simulink model "ControlSystemPID"  (R2020b)
settings: Solver=ode23s  StartTime=0.0  StopTime=3.5  MaxStep=0.06  RelTol=1e-3
model workspace: external: MATLAB File C:\Users\User\Aalborg Universitet\ROB 3 - General\P3\Solidworks_files\SimScapeV4\TotalAssemblyV4_DataFile.m (data not in the file)
values from neighbouring files (symbols this model uses):
  Ki = 10    [Data.m]
  Kp = 200    [Data.m]
  Kv = 127    [Data.m]
undefined symbols (not defined in the file or in its folder): smiData, X, Y, Z
libraries: sm_lib x112, nesl_utility x16, simulink_extras x9, pid_lib x1
(part 3 of 3)

== system ControlSystemPID/Body3_3_RIGID/Finger_2_RIGID ==
  ReferenceFrame : sm_lib/Frames and Transforms/Reference Frame
  Solid : sm_lib/Body Elements/File Solid  ExtGeomFileName=Finger_Default_sldprt.STEP  UnitType=FromFile  ExtGeomFileUnits=m  StepReaderType=HEX  ExportConvexHullGeometry=off  InertiaType=Custom  Mass=smiData.Solid(16).mass  MassUnits=kg  CenterOfMass=smiData.Solid(16).CoM  CenterOfMassUnits=mm  MomentsOfInertia=smiData.Solid(16).MoI  MomentsOfInertiaUnits=kg*mm^2  ProductsOfInertia=smiData.Solid(16).PoI  ProductsOfInertiaUnits=kg*mm^2  BasedOnType=DensityFromFile  Density=1000  DensityUnits=kg/m^3  DoExposeReferenceFrame=on  SerializedFrames=<Frames/>  GraphicType=FromGeometry  MarkerShape=Sphere  MarkerSize=10  GraphicVisPropType=SimpleVisualProperties  GraphicDiffuseColor=smiData.Solid(16).color  GraphicSpecularColor=[0.5 0.5 0.5 1.0]  GraphicAmbientColor=[0.15 0.15 0.15 1.0]  GraphicEmissiveColor=[0.0 0.0 0.0 1.0]  GraphicShininess=75  GraphicOpacity=smiData.Solid(16).opacity
  F : PMIOPort  Side=Left
  connections:
  Solid/RConn1 -- ReferenceFrame/RConn1 -- F/RConn1

== system ControlSystemPID/Body3_3_RIGID/Link_2_1_RIGID ==
  ReferenceFrame : sm_lib/Frames and Transforms/Reference Frame
  Solid : sm_lib/Body Elements/File Solid  ExtGeomFileName=Link-2_Default_sldprt.STEP  UnitType=FromFile  ExtGeomFileUnits=m  StepReaderType=HEX  ExportConvexHullGeometry=off  InertiaType=Custom  Mass=smiData.Solid(11).mass  MassUnits=kg  CenterOfMass=smiData.Solid(11).CoM  CenterOfMassUnits=mm  MomentsOfInertia=smiData.Solid(11).MoI  MomentsOfInertiaUnits=kg*mm^2  ProductsOfInertia=smiData.Solid(11).PoI  ProductsOfInertiaUnits=kg*mm^2  BasedOnType=DensityFromFile  Density=1000  DensityUnits=kg/m^3  DoExposeReferenceFrame=on  SerializedFrames=<Frames/>  GraphicType=FromGeometry  MarkerShape=Sphere  MarkerSize=10  GraphicVisPropType=SimpleVisualProperties  GraphicDiffuseColor=smiData.Solid(11).color  GraphicSpecularColor=[0.5 0.5 0.5 1.0]  GraphicAmbientColor=[0.15 0.15 0.15 1.0]  GraphicEmissiveColor=[0.0 0.0 0.0 1.0]  GraphicShininess=75  GraphicOpacity=smiData.Solid(11).opacity
  F : PMIOPort  Side=Left
  connections:
  Solid/RConn1 -- ReferenceFrame/RConn1 -- F/RConn1

== system ControlSystemPID/Body3_3_RIGID/Link_plate_1_RIGID ==
  ReferenceFrame : sm_lib/Frames and Transforms/Reference Frame
  Solid : sm_lib/Body Elements/File Solid  ExtGeomFileName=Link-plate_Default_sldprt.STEP  UnitType=FromFile  ExtGeomFileUnits=m  StepReaderType=HEX  ExportConvexHullGeometry=off  InertiaType=Custom  Mass=smiData.Solid(3).mass  MassUnits=kg  CenterOfMass=smiData.Solid(3).CoM  CenterOfMassUnits=mm  MomentsOfInertia=smiData.Solid(3).MoI  MomentsOfInertiaUnits=kg*mm^2  ProductsOfInertia=smiData.Solid(3).PoI  ProductsOfInertiaUnits=kg*mm^2  BasedOnType=DensityFromFile  Density=1000  DensityUnits=kg/m^3  DoExposeReferenceFrame=on  SerializedFrames=<Frames/>  GraphicType=FromGeometry  MarkerShape=Sphere  MarkerSize=10  GraphicVisPropType=SimpleVisualProperties  GraphicDiffuseColor=smiData.Solid(3).color  GraphicSpecularColor=[0.5 0.5 0.5 1.0]  GraphicAmbientColor=[0.15 0.15 0.15 1.0]  GraphicEmissiveColor=[0.0 0.0 0.0 1.0]  GraphicShininess=75  GraphicOpacity=smiData.Solid(3).opacity
  F : PMIOPort  Side=Left
  connections:
  Solid/RConn1 -- ReferenceFrame/RConn1 -- F/RConn1

== system ControlSystemPID/Body3_3_RIGID/MX_28T_1_RIGID ==
  ReferenceFrame : sm_lib/Frames and Transforms/Reference Frame
  Solid : sm_lib/Body Elements/File Solid  ExtGeomFileName=MX-28T_Default_sldprt.STEP  UnitType=FromFile  ExtGeomFileUnits=m  StepReaderType=HEX  ExportConvexHullGeometry=off  InertiaType=Custom  Mass=smiData.Solid(13).mass  MassUnits=kg  CenterOfMass=smiData.Solid(13).CoM  CenterOfMassUnits=mm  MomentsOfInertia=smiData.Solid(13).MoI  MomentsOfInertiaUnits=kg*mm^2  ProductsOfInertia=smiData.Solid(13).PoI  ProductsOfInertiaUnits=kg*mm^2  BasedOnType=DensityFromFile  Density=1000  DensityUnits=kg/m^3  DoExposeReferenceFrame=on  SerializedFrames=<Frames/>  GraphicType=FromGeometry  MarkerShape=Sphere  MarkerSize=10  GraphicVisPropType=SimpleVisualProperties  GraphicDiffuseColor=smiData.Solid(13).color  GraphicSpecularColor=[0.5 0.5 0.5 1.0]  GraphicAmbientColor=[0.15 0.15 0.15 1.0]  GraphicEmissiveColor=[0.0 0.0 0.0 1.0]  GraphicShininess=75  GraphicOpacity=smiData.Solid(13).opacity
  F : PMIOPort  Side=Left
  connections:
  Solid/RConn1 -- ReferenceFrame/RConn1 -- F/RConn1

== system ControlSystemPID/Body3_3_RIGID/MX_28T_2_RIGID ==
  ReferenceFrame : sm_lib/Frames and Transforms/Reference Frame
  Solid : sm_lib/Body Elements/File Solid  ExtGeomFileName=MX-28T_Default_sldprt.STEP  UnitType=FromFile  ExtGeomFileUnits=m  StepReaderType=HEX  ExportConvexHullGeometry=off  InertiaType=Custom  Mass=smiData.Solid(13).mass  MassUnits=kg  CenterOfMass=smiData.Solid(13).CoM  CenterOfMassUnits=mm  MomentsOfInertia=smiData.Solid(13).MoI  MomentsOfInertiaUnits=kg*mm^2  ProductsOfInertia=smiData.Solid(13).PoI  ProductsOfInertiaUnits=kg*mm^2  BasedOnType=DensityFromFile  Density=1000  DensityUnits=kg/m^3  DoExposeReferenceFrame=on  SerializedFrames=<Frames/>  GraphicType=FromGeometry  MarkerShape=Sphere  MarkerSize=10  GraphicVisPropType=SimpleVisualProperties  GraphicDiffuseColor=smiData.Solid(13).color  GraphicSpecularColor=[0.5 0.5 0.5 1.0]  GraphicAmbientColor=[0.15 0.15 0.15 1.0]  GraphicEmissiveColor=[0.0 0.0 0.0 1.0]  GraphicShininess=75  GraphicOpacity=smiData.Solid(13).opacity
  F : PMIOPort  Side=Left
  connections:
  Solid/RConn1 -- ReferenceFrame/RConn1 -- F/RConn1

== system ControlSystemPID/Body3_3_RIGID/MX_28T_Link_1_RIGID ==
  ReferenceFrame : sm_lib/Frames and Transforms/Reference Frame
  Solid : sm_lib/Body Elements/File Solid  ExtGeomFileName=MX-28T-Link_Default_sldprt.STEP  UnitType=FromFile  ExtGeomFileUnits=m  StepReaderType=HEX  ExportConvexHullGeometry=off  InertiaType=Custom  Mass=smiData.Solid(17).mass  MassUnits=kg  CenterOfMass=smiData.Solid(17).CoM  CenterOfMassUnits=mm  MomentsOfInertia=smiData.Solid(17).MoI  MomentsOfInertiaUnits=kg*mm^2  ProductsOfInertia=smiData.Solid(17).PoI  ProductsOfInertiaUnits=kg*mm^2  BasedOnType=DensityFromFile  Density=1000  DensityUnits=kg/m^3  DoExposeReferenceFrame=on  SerializedFrames=<Frames/>  GraphicType=FromGeometry  MarkerShape=Sphere  MarkerSize=10  GraphicVisPropType=SimpleVisualProperties  GraphicDiffuseColor=smiData.Solid(17).color  GraphicSpecularColor=[0.5 0.5 0.5 1.0]  GraphicAmbientColor=[0.15 0.15 0.15 1.0]  GraphicEmissiveColor=[0.0 0.0 0.0 1.0]  GraphicShininess=75  GraphicOpacity=smiData.Solid(17).opacity
  F : PMIOPort  Side=Left
  connections:
  Solid/RConn1 -- ReferenceFrame/RConn1 -- F/RConn1

== system ControlSystemPID/Body3_3_RIGID/MX_28T_Link_2_RIGID ==
  ReferenceFrame : sm_lib/Frames and Transforms/Reference Frame
  Solid : sm_lib/Body Elements/File Solid  ExtGeomFileName=MX-28T-Link_Default_sldprt.STEP  UnitType=FromFile  ExtGeomFileUnits=m  StepReaderType=HEX  ExportConvexHullGeometry=off  InertiaType=Custom  Mass=smiData.Solid(17).mass  MassUnits=kg  CenterOfMass=smiData.Solid(17).CoM  CenterOfMassUnits=mm  MomentsOfInertia=smiData.Solid(17).MoI  MomentsOfInertiaUnits=kg*mm^2  ProductsOfInertia=smiData.Solid(17).PoI  ProductsOfInertiaUnits=kg*mm^2  BasedOnType=DensityFromFile  Density=1000  DensityUnits=kg/m^3  DoExposeReferenceFrame=on  SerializedFrames=<Frames/>  GraphicType=FromGeometry  MarkerShape=Sphere  MarkerSize=10  GraphicVisPropType=SimpleVisualProperties  GraphicDiffuseColor=smiData.Solid(17).color  GraphicSpecularColor=[0.5 0.5 0.5 1.0]  GraphicAmbientColor=[0.15 0.15 0.15 1.0]  GraphicEmissiveColor=[0.0 0.0 0.0 1.0]  GraphicShininess=75  GraphicOpacity=smiData.Solid(17).opacity
  F : PMIOPort  Side=Left
  connections:
  Solid/RConn1 -- ReferenceFrame/RConn1 -- F/RConn1

== system ControlSystemPID/Body3_3_RIGID/Servo_Disc_1_RIGID ==
  ReferenceFrame : sm_lib/Frames and Transforms/Reference Frame
  Solid : sm_lib/Body Elements/File Solid  ExtGeomFileName=Servo-Disc_Default_sldprt.STEP  UnitType=FromFile  ExtGeomFileUnits=m  StepReaderType=HEX  ExportConvexHullGeometry=off  InertiaType=Custom  Mass=smiData.Solid(2).mass  MassUnits=kg  CenterOfMass=smiData.Solid(2).CoM  CenterOfMassUnits=mm  MomentsOfInertia=smiData.Solid(2).MoI  MomentsOfInertiaUnits=kg*mm^2  ProductsOfInertia=smiData.Solid(2).PoI  ProductsOfInertiaUnits=kg*mm^2  BasedOnType=DensityFromFile  Density=1000  DensityUnits=kg/m^3  DoExposeReferenceFrame=on  SerializedFrames=<Frames/>  GraphicType=FromGeometry  MarkerShape=Sphere  MarkerSize=10  GraphicVisPropType=SimpleVisualProperties  GraphicDiffuseColor=smiData.Solid(2).color  GraphicSpecularColor=[0.5 0.5 0.5 1.0]  GraphicAmbientColor=[0.15 0.15 0.15 1.0]  GraphicEmissiveColor=[0.0 0.0 0.0 1.0]  GraphicShininess=75  GraphicOpacity=smiData.Solid(2).opacity
  F : PMIOPort  Side=Left
  connections:
  Solid/RConn1 -- ReferenceFrame/RConn1 -- F/RConn1

== system ControlSystemPID/Body3_3_RIGID/Servo_Disc_2_RIGID ==
  ReferenceFrame : sm_lib/Frames and Transforms/Reference Frame
  Solid : sm_lib/Body Elements/File Solid  ExtGeomFileName=Servo-Disc_Default_sldprt.STEP  UnitType=FromFile  ExtGeomFileUnits=m  StepReaderType=HEX  ExportConvexHullGeometry=off  InertiaType=Custom  Mass=smiData.Solid(2).mass  MassUnits=kg  CenterOfMass=smiData.Solid(2).CoM  CenterOfMassUnits=mm  MomentsOfInertia=smiData.Solid(2).MoI  MomentsOfInertiaUnits=kg*mm^2  ProductsOfInertia=smiData.Solid(2).PoI  ProductsOfInertiaUnits=kg*mm^2  BasedOnType=DensityFromFile  Density=1000  DensityUnits=kg/m^3  DoExposeReferenceFrame=on  SerializedFrames=<Frames/>  GraphicType=FromGeometry  MarkerShape=Sphere  MarkerSize=10  GraphicVisPropType=SimpleVisualProperties  GraphicDiffuseColor=smiData.Solid(2).color  GraphicSpecularColor=[0.5 0.5 0.5 1.0]  GraphicAmbientColor=[0.15 0.15 0.15 1.0]  GraphicEmissiveColor=[0.0 0.0 0.0 1.0]  GraphicShininess=75  GraphicOpacity=smiData.Solid(2).opacity
  F : PMIOPort  Side=Left
  connections:
  Solid/RConn1 -- ReferenceFrame/RConn1 -- F/RConn1

== system ControlSystemPID/Body3_3_RIGID/Servo_Disc_3_RIGID ==
  ReferenceFrame : sm_lib/Frames and Transforms/Reference Frame
  Solid : sm_lib/Body Elements/File Solid  ExtGeomFileName=Servo-Disc_Default_sldprt.STEP  UnitType=FromFile  ExtGeomFileUnits=m  StepReaderType=HEX  ExportConvexHullGeometry=off  InertiaType=Custom  Mass=smiData.Solid(2).mass  MassUnits=kg  CenterOfMass=smiData.Solid(2).CoM  CenterOfMassUnits=mm  MomentsOfInertia=smiData.Solid(2).MoI  MomentsOfInertiaUnits=kg*mm^2  ProductsOfInertia=smiData.Solid(2).PoI  ProductsOfInertiaUnits=kg*mm^2  BasedOnType=DensityFromFile  Density=1000  DensityUnits=kg/m^3  DoExposeReferenceFrame=on  SerializedFrames=<Frames/>  GraphicType=FromGeometry  MarkerShape=Sphere  MarkerSize=10  GraphicVisPropType=SimpleVisualProperties  GraphicDiffuseColor=smiData.Solid(2).color  GraphicSpecularColor=[0.5 0.5 0.5 1.0]  GraphicAmbientColor=[0.15 0.15 0.15 1.0]  GraphicEmissiveColor=[0.0 0.0 0.0 1.0]  GraphicShininess=75  GraphicOpacity=smiData.Solid(2).opacity
  F : PMIOPort  Side=Left
  connections:
  Solid/RConn1 -- ReferenceFrame/RConn1 -- F/RConn1

== system ControlSystemPID/Body3_3_RIGID/Servo_Disc_4_RIGID ==
  ReferenceFrame : sm_lib/Frames and Transforms/Reference Frame
  Solid : sm_lib/Body Elements/File Solid  ExtGeomFileName=Servo-Disc_Default_sldprt.STEP  UnitType=FromFile  ExtGeomFileUnits=m  StepReaderType=HEX  ExportConvexHullGeometry=off  InertiaType=Custom  Mass=smiData.Solid(2).mass  MassUnits=kg  CenterOfMass=smiData.Solid(2).CoM  CenterOfMassUnits=mm  MomentsOfInertia=smiData.Solid(2).MoI  MomentsOfInertiaUnits=kg*mm^2  ProductsOfInertia=smiData.Solid(2).PoI  ProductsOfInertiaUnits=kg*mm^2  BasedOnType=DensityFromFile  Density=1000  DensityUnits=kg/m^3  DoExposeReferenceFrame=on  SerializedFrames=<Frames/>  GraphicType=FromGeometry  MarkerShape=Sphere  MarkerSize=10  GraphicVisPropType=SimpleVisualProperties  GraphicDiffuseColor=smiData.Solid(2).color  GraphicSpecularColor=[0.5 0.5 0.5 1.0]  GraphicAmbientColor=[0.15 0.15 0.15 1.0]  GraphicEmissiveColor=[0.0 0.0 0.0 1.0]  GraphicShininess=75  GraphicOpacity=smiData.Solid(2).opacity
  F : PMIOPort  Side=Left
  connections:
  Solid/RConn1 -- ReferenceFrame/RConn1 -- F/RConn1

== system ControlSystemPID/Body3_3_RIGID/Servo_Disc_5_RIGID ==
  ReferenceFrame : sm_lib/Frames and Transforms/Reference Frame
  Solid : sm_lib/Body Elements/File Solid  ExtGeomFileName=Servo-Disc_Default_sldprt.STEP  UnitType=FromFile  ExtGeomFileUnits=m  StepReaderType=HEX  ExportConvexHullGeometry=off  InertiaType=Custom  Mass=smiData.Solid(2).mass  MassUnits=kg  CenterOfMass=smiData.Solid(2).CoM  CenterOfMassUnits=mm  MomentsOfInertia=smiData.Solid(2).MoI  MomentsOfInertiaUnits=kg*mm^2  ProductsOfInertia=smiData.Solid(2).PoI  ProductsOfInertiaUnits=kg*mm^2  BasedOnType=DensityFromFile  Density=1000  DensityUnits=kg/m^3  DoExposeReferenceFrame=on  SerializedFrames=<Frames/>  GraphicType=FromGeometry  MarkerShape=Sphere  MarkerSize=10  GraphicVisPropType=SimpleVisualProperties  GraphicDiffuseColor=smiData.Solid(2).color  GraphicSpecularColor=[0.5 0.5 0.5 1.0]  GraphicAmbientColor=[0.15 0.15 0.15 1.0]  GraphicEmissiveColor=[0.0 0.0 0.0 1.0]  GraphicShininess=75  GraphicOpacity=smiData.Solid(2).opacity
  F : PMIOPort  Side=Left
  connections:
  Solid/RConn1 -- ReferenceFrame/RConn1 -- F/RConn1

== system ControlSystemPID/Body3_3_RIGID/Servo_Disc_6_RIGID ==
  ReferenceFrame : sm_lib/Frames and Transforms/Reference Frame
  Solid : sm_lib/Body Elements/File Solid  ExtGeomFileName=Servo-Disc_Default_sldprt.STEP  UnitType=FromFile  ExtGeomFileUnits=m  StepReaderType=HEX  ExportConvexHullGeometry=off  InertiaType=Custom  Mass=smiData.Solid(2).mass  MassUnits=kg  CenterOfMass=smiData.Solid(2).CoM  CenterOfMassUnits=mm  MomentsOfInertia=smiData.Solid(2).MoI  MomentsOfInertiaUnits=kg*mm^2  ProductsOfInertia=smiData.Solid(2).PoI  ProductsOfInertiaUnits=kg*mm^2  BasedOnType=DensityFromFile  Density=1000  DensityUnits=kg/m^3  DoExposeReferenceFrame=on  SerializedFrames=<Frames/>  GraphicType=FromGeometry  MarkerShape=Sphere  MarkerSize=10  GraphicVisPropType=SimpleVisualProperties  GraphicDiffuseColor=smiData.Solid(2).color  GraphicSpecularColor=[0.5 0.5 0.5 1.0]  GraphicAmbientColor=[0.15 0.15 0.15 1.0]  GraphicEmissiveColor=[0.0 0.0 0.0 1.0]  GraphicShininess=75  GraphicOpacity=smiData.Solid(2).opacity
  F : PMIOPort  Side=Left
  connections:
  Solid/RConn1 -- ReferenceFrame/RConn1 -- F/RConn1

== system ControlSystemPID/Body3_3_RIGID/Servo_disc_link_MX_28T_1_RIGID ==
  ReferenceFrame : sm_lib/Frames and Transforms/Reference Frame
  Solid : sm_lib/Body Elements/File Solid  ExtGeomFileName=Servo-disc-link_MX-28T_Default_sldprt.STEP  UnitType=FromFile  ExtGeomFileUnits=m  StepReaderType=HEX  ExportConvexHullGeometry=off  InertiaType=Custom  Mass=smiData.Solid(15).mass  MassUnits=kg  CenterOfMass=smiData.Solid(15).CoM  CenterOfMassUnits=mm  MomentsOfInertia=smiData.Solid(15).MoI  MomentsOfInertiaUnits=kg*mm^2  ProductsOfInertia=smiData.Solid(15).PoI  ProductsOfInertiaUnits=kg*mm^2  BasedOnType=DensityFromFile  Density=1000  DensityUnits=kg/m^3  DoExposeReferenceFrame=on  SerializedFrames=<Frames/>  GraphicType=FromGeometry  MarkerShape=Sphere  MarkerSize=10  GraphicVisPropType=SimpleVisualProperties  GraphicDiffuseColor=smiData.Solid(15).color  GraphicSpecularColor=[0.5 0.5 0.5 1.0]  GraphicAmbientColor=[0.15 0.15 0.15 1.0]  GraphicEmissiveColor=[0.0 0.0 0.0 1.0]  GraphicShininess=75  GraphicOpacity=smiData.Solid(15).opacity
  F : PMIOPort  Side=Left
  connections:
  Solid/RConn1 -- ReferenceFrame/RConn1 -- F/RConn1

== system ControlSystemPID/Body3_3_RIGID/Servo_disc_link_MX_28T_2_RIGID ==
  ReferenceFrame : sm_lib/Frames and Transforms/Reference Frame
  Solid : sm_lib/Body Elements/File Solid  ExtGeomFileName=Servo-disc-link_MX-28T_Default_sldprt.STEP  UnitType=FromFile  ExtGeomFileUnits=m  StepReaderType=HEX  ExportConvexHullGeometry=off  InertiaType=Custom  Mass=smiData.Solid(15).mass  MassUnits=kg  CenterOfMass=smiData.Solid(15).CoM  CenterOfMassUnits=mm  MomentsOfInertia=smiData.Solid(15).MoI  MomentsOfInertiaUnits=kg*mm^2  ProductsOfInertia=smiData.Solid(15).PoI  ProductsOfInertiaUnits=kg*mm^2  BasedOnType=DensityFromFile  Density=1000  DensityUnits=kg/m^3  DoExposeReferenceFrame=on  SerializedFrames=<Frames/>  GraphicType=FromGeometry  MarkerShape=Sphere  MarkerSize=10  GraphicVisPropType=SimpleVisualProperties  GraphicDiffuseColor=smiData.Solid(15).color  GraphicSpecularColor=[0.5 0.5 0.5 1.0]  GraphicAmbientColor=[0.15 0.15 0.15 1.0]  GraphicEmissiveColor=[0.0 0.0 0.0 1.0]  GraphicShininess=75  GraphicOpacity=smiData.Solid(15).opacity
  F : PMIOPort  Side=Left
  connections:
  Solid/RConn1 -- ReferenceFrame/RConn1 -- F/RConn1

== system ControlSystemPID/Body3_3_RIGID/Servo_disc_link_MX_64T_1_RIGID ==
  ReferenceFrame : sm_lib/Frames and Transforms/Reference Frame
  Solid : sm_lib/Body Elements/File Solid  ExtGeomFileName=Servo-disc-link_MX-64T_Default_sldprt.STEP  UnitType=FromFile  ExtGeomFileUnits=m  StepReaderType=HEX  ExportConvexHullGeometry=off  InertiaType=Custom  Mass=smiData.Solid(12).mass  MassUnits=kg  CenterOfMass=smiData.Solid(12).CoM  CenterOfMassUnits=mm  MomentsOfInertia=smiData.Solid(12).MoI  MomentsOfInertiaUnits=kg*mm^2  ProductsOfInertia=smiData.Solid(12).PoI  ProductsOfInertiaUnits=kg*mm^2  BasedOnType=DensityFromFile  Density=1000  DensityUnits=kg/m^3  DoExposeReferenceFrame=on  SerializedFrames=<Frames/>  GraphicType=FromGeometry  MarkerShape=Sphere  MarkerSize=10  GraphicVisPropType=SimpleVisualProperties  GraphicDiffuseColor=smiData.Solid(12).color  GraphicSpecularColor=[0.5 0.5 0.5 1.0]  GraphicAmbientColor=[0.15 0.15 0.15 1.0]  GraphicEmissiveColor=[0.0 0.0 0.0 1.0]  GraphicShininess=75  GraphicOpacity=smiData.Solid(12).opacity
  F : PMIOPort  Side=Left
  connections:
  Solid/RConn1 -- ReferenceFrame/RConn1 -- F/RConn1

== system ControlSystemPID/Body3_3_RIGID/Servo_link_link_MX_28T_4_RIGID ==
  ReferenceFrame : sm_lib/Frames and Transforms/Reference Frame
  Solid : sm_lib/Body Elements/File Solid  ExtGeomFileName=Servo-link-link_MX-28T_Default_sldprt.STEP  UnitType=FromFile  ExtGeomFileUnits=m  StepReaderType=HEX  ExportConvexHullGeometry=off  InertiaType=Custom  Mass=smiData.Solid(14).mass  MassUnits=kg  CenterOfMass=smiData.Solid(14).CoM  CenterOfMassUnits=mm  MomentsOfInertia=smiData.Solid(14).MoI  MomentsOfInertiaUnits=kg*mm^2  ProductsOfInertia=smiData.Solid(14).PoI  ProductsOfInertiaUnits=kg*mm^2  BasedOnType=DensityFromFile  Density=1000  DensityUnits=kg/m^3  DoExposeReferenceFrame=on  SerializedFrames=<Frames/>  GraphicType=FromGeometry  MarkerShape=Sphere  MarkerSize=10  GraphicVisPropType=SimpleVisualProperties  GraphicDiffuseColor=smiData.Solid(14).color  GraphicSpecularColor=[0.5 0.5 0.5 1.0]  GraphicAmbientColor=[0.15 0.15 0.15 1.0]  GraphicEmissiveColor=[0.0 0.0 0.0 1.0]  GraphicShininess=75  GraphicOpacity=smiData.Solid(14).opacity
  F : PMIOPort  Side=Left
  connections:
  Solid/RConn1 -- ReferenceFrame/RConn1 -- F/RConn1

== system ControlSystemPID/TableAssembly_2_RIGID/Base_1_RIGID ==
  ReferenceFrame : sm_lib/Frames and Transforms/Reference Frame
  Solid : sm_lib/Body Elements/File Solid  ExtGeomFileName=Base_Default_sldprt.STEP  UnitType=FromFile  ExtGeomFileUnits=m  StepReaderType=HEX  ExportConvexHullGeometry=off  InertiaType=Custom  Mass=smiData.Solid(7).mass  MassUnits=kg  CenterOfMass=smiData.Solid(7).CoM  CenterOfMassUnits=mm  MomentsOfInertia=smiData.Solid(7).MoI  MomentsOfInertiaUnits=kg*mm^2  ProductsOfInertia=smiData.Solid(7).PoI  ProductsOfInertiaUnits=kg*mm^2  BasedOnType=DensityFromFile  Density=1000  DensityUnits=kg/m^3  DoExposeReferenceFrame=on  SerializedFrames=<Frames/>  GraphicType=FromGeometry  MarkerShape=Sphere  MarkerSize=10  GraphicVisPropType=SimpleVisualProperties  GraphicDiffuseColor=smiData.Solid(7).color  GraphicSpecularColor=[0.5 0.5 0.5 1.0]  GraphicAmbientColor=[0.15 0.15 0.15 1.0]  GraphicEmissiveColor=[0.0 0.0 0.0 1.0]  GraphicShininess=75  GraphicOpacity=smiData.Solid(7).opacity
  F : PMIOPort  Side=Left
  connections:
  Solid/RConn1 -- ReferenceFrame/RConn1 -- F/RConn1

== system ControlSystemPID/TableAssembly_2_RIGID/MX_64T_1_RIGID ==
  ReferenceFrame : sm_lib/Frames and Transforms/Reference Frame
  Solid : sm_lib/Body Elements/File Solid  ExtGeomFileName=MX-64T_Default_sldprt.STEP  UnitType=FromFile  ExtGeomFileUnits=m  StepReaderType=HEX  ExportConvexHullGeometry=off  InertiaType=Custom  Mass=smiData.Solid(1).mass  MassUnits=kg  CenterOfMass=smiData.Solid(1).CoM  CenterOfMassUnits=mm  MomentsOfInertia=smiData.Solid(1).MoI  MomentsOfInertiaUnits=kg*mm^2  ProductsOfInertia=smiData.Solid(1).PoI  ProductsOfInertiaUnits=kg*mm^2  BasedOnType=DensityFromFile  Density=1000  DensityUnits=kg/m^3  DoExposeReferenceFrame=on  SerializedFrames=<Frames/>  GraphicType=FromGeometry  MarkerShape=Sphere  MarkerSize=10  GraphicVisPropType=SimpleVisualProperties  GraphicDiffuseColor=smiData.Solid(1).color  GraphicSpecularColor=[0.5 0.5 0.5 1.0]  GraphicAmbientColor=[0.15 0.15 0.15 1.0]  GraphicEmissiveColor=[0.0 0.0 0.0 1.0]  GraphicShininess=75  GraphicOpacity=smiData.Solid(1).opacity
  F : PMIOPort  Side=Left
  connections:
  Solid/RConn1 -- ReferenceFrame/RConn1 -- F/RConn1

== matlab function ControlSystemPID/Joint 2/MATLAB Function3 ==
  data: ddtheta input; output output; Verror input; Perror input; PiError input; Kp input; Kv input; Ki input
function output = PID(ddtheta, Verror, Perror, PiError,Kp,Kv,Ki)

output = ddtheta+Kv*Verror+Kp*Perror+Ki*PiError;

== matlab function ControlSystemPID/Joint 2/MATLAB Function4 ==
  data: ddtheta input; output output; Verror input; Perror input; PiError input; Kp input; Kv input; Ki input
function output = PID(ddtheta, Verror, Perror, PiError,Kp,Kv,Ki)

output = ddtheta+Kv*Verror+Kp*Perror+Ki*PiError;

== matlab function ControlSystemPID/Joint 1/MATLAB Function ==
  data: ddtheta1 input; MTau1 output; theta2 input; ddtheta2 input; theta3 input; ddtheta3 input
function MTau1  = MassMatrix(ddtheta1,theta2,ddtheta2, theta3,ddtheta3)

MTau1=ddtheta2*(0.000032669184954733717964837201853562*cos(theta2 + theta3 + 1.569333479860983395711863672254) - 0.000017807919999999997375493554496728*sin(theta2)) + 0.000032669184954733717964837201853562*ddtheta3*cos(theta2 + theta3 + 1.569333479860983395711863672254) + ddtheta1*(0.00028211582749044971299237401724541*cos(2.0*theta2 + 2.0*theta3 - 0.00025333566500056721070216563328695) - 0.0066126117710137419890825584183635*cos(2.0*theta2 - 0.001752443109112493633835037904297) - 0.0088297863675000001076886846362868*cos(2.0*theta2 + theta3) + 0.0088297863675000001076886846362868*cos(theta3) + 0.020477058988725500149330471799658);
end

== matlab function ControlSystemPID/Joint 1/MATLAB Function1 ==
  data: theta1 input; VGTau1 output; dtheta1 input; theta2 input; dtheta2 input; theta3 input; dtheta3 input
function VGTau1 = VelocityGravity(theta1,dtheta1,theta2,dtheta2, theta3,dtheta3)
g =-9.82;
G=0;
V=0.000045525453907039893077998704562503*dtheta2^2*sin(2.0*theta2 - 0.069813170079773183076947630739545*theta1) - 0.000045525453907039893077998704562503*dtheta2^2*sin(0.069813170079773183076947630739545*theta1 + 2.0*theta2) + 0.000012256666221467139594319961659608*dtheta2^2*sin(2.0*theta2 - 0.069813170079773183076947630739545*theta1 + 2.0*theta3) - 0.000012256666221467139594319961659608*dtheta2^2*sin(0.069813170079773183076947630739545*theta1 + 2.0*theta2 + 2.0*theta3) + 0.000012256666221467139594319961659608*dtheta3^2*sin(2.0*theta2 - 0.069813170079773183076947630739545*theta1 + 2.0*theta3) - 0.000012256666221467139594319961659608*dtheta3^2*sin(0.069813170079773183076947630739545*theta1 + 2.0*theta2 + 2.0*theta3) + 0.000038527211090146256733997981447359*dtheta2^2*sin(theta3 - 0.069813170079773183076947630739545*theta1) - 0.000038527211090146256733997981447359*dtheta2^2*sin(0.069813170079773183076947630739545*theta1 + theta3) + 0.000038527211090146256733997981447359*dtheta2^2*sin(2.0*theta2 - 0.069813170079773183076947630739545*theta1 + theta3) - 0.000038527211090146256733997981447359*dtheta2^2*sin(0.069813170079773183076947630739545*theta1 + 2.0*theta2 + theta3) - 0.00011556424025701406534463733244422*dtheta2^2*sin(0.069813170079773183076947630739545*theta1) - 0.000024513332442934279188639923319215*dtheta3^2*sin(0.069813170079773183076947630739545*theta1) - 0.000032669149999999998743634849196482*dtheta2^2*cos(theta2 + theta3) - 0.000032669149999999998743634849196482*dtheta3^2*cos(theta2 + theta3) - 0.000000047789999999999999785588042843995*dtheta2^2*sin(theta2 + theta3) - 0.000000047789999999999999785588042843995*dtheta3^2*sin(theta2 + theta3) - 0.000017807919999999997375493554496728*dtheta2^2*cos(theta2) - 0.0088297863675000001076886846362868*dtheta1*dtheta3*sin(theta3) + 0.00000014294000000000000807948597348479*dtheta1*dtheta2*cos(2.0*theta2 + 2.0*theta3) + 0.00000014294000000000000807948597348479*dtheta1*dtheta3*cos(2.0*theta2 + 2.0*theta3) - 0.00056423163687499935155938990405389*dtheta1*dtheta2*sin(2.0*theta2 + 2.0*theta3) - 0.00056423163687499935155938990405389*dtheta1*dtheta3*sin(2.0*theta2 + 2.0*theta3) + 0.000024513332442934279188639923319215*dtheta2*dtheta3*sin(2.0*theta2 - 0.069813170079773183076947630739545*theta1 + 2.0*theta3) - 0.000024513332442934279188639923319215*dtheta2*dtheta3*sin(0.069813170079773183076947630739545*theta1 + 2.0*theta2 + 2.0*theta3) + 0.017659572735000000215377369272574*dtheta1*dtheta2*sin(2.0*theta2 + theta3) + 0.0088297863675000001076886846362868*dtheta1*dtheta3*sin(2.0*theta2 + theta3) + 0.000038527211090146256733997981447359*dtheta2*dtheta3*sin(theta3 - 0.069813170079773183076947630739545*theta1) - 0.000038527211090146256733997981447359*dtheta2*dtheta3*sin(0.069813170079773183076947630739545*theta1 + theta3) + 0.000038527211090146256733997981447359*dtheta2*dtheta3*sin(2.0*theta2 - 0.069813170079773183076947630739545*theta1 + theta3) - 0.000038527211090146256733997981447359*dtheta2*dtheta3*sin(0.069813170079773183076947630739545*theta1 + 2.0*theta2 + theta3) - 0.000023176439999999999975327513723755*dtheta1*dtheta2*cos(2.0*theta2) + 0.013225203234326000922838062479059*dtheta1*dtheta2*sin(2.0*theta2) - 0.00004902666488586855837727984663843*dtheta2*dtheta3*sin(0.069813170079773183076947630739545*theta1) - 0.000065338299999999997487269698392964*dtheta2*dtheta3*cos(theta2 + theta3) - 0.00000009557999999999999957117608568799*dtheta2*dtheta3*sin(theta2 + theta3);
VGTau1=V+G;
end

== matlab function ControlSystemPID/Joint 1/MATLAB Function2 ==
  data: ddtheta input; output output; Verror input; Perror input; PiError input; Kp input; Kv input; Ki input
function output = PID(ddtheta, Verror, Perror, PiError,Kp,Kv,Ki)

output = ddtheta+Kv*Verror+Kp*Perror+Ki*PiError;

== matlab function ControlSystemPID/Joint 1/MATLAB Function3 ==
  data: ddtheta input; output output; Verror input; Perror input; PiError input; Kp input; Kv input; Ki input
function output = PID(ddtheta, Verror, Perror, PiError,Kp,Kv,Ki)

output = ddtheta+Kv*Verror+Kp*Perror+Ki*PiError;

== matlab function ControlSystemPID/Joint 1/MATLAB Function4 ==
  data: ddtheta input; output output; Verror input; Perror input; PiError input; Kp input; Kv input; Ki input
function output = PID(ddtheta, Verror, Perror, PiError,Kp,Kv,Ki)

output = ddtheta+Kv*Verror+Kp*Perror+Ki*PiError;

== matlab function ControlSystemPID/Joint 3/MATLAB Function2 ==
  data: ddtheta input; output output; Verror input; Perror input; PiError input; Kp input; Kv input; Ki input
function output = PID(ddtheta, Verror, Perror, PiError,Kp,Kv,Ki)

output = ddtheta+Kv*Verror+Kp*Perror+Ki*PiError;

== matlab function ControlSystemPID/Joint 3/MATLAB Function3 ==
  data: ddtheta input; output output; Verror input; Perror input; PiError input; Kp input; Kv input; Ki input
function output = PID(ddtheta, Verror, Perror, PiError,Kp,Kv,Ki)

output = ddtheta+Kv*Verror+Kp*Perror+Ki*PiError;

== matlab function ControlSystemPID/Joint 3/MATLAB Function4 ==
  data: ddtheta input; output output; Verror input; Perror input; PiError input; Kp input; Kv input; Ki input
function output = PID(ddtheta, Verror, Perror, PiError,Kp,Kv,Ki)

output = ddtheta+Kv*Verror+Kp*Perror+Ki*PiError;

== matlab function ControlSystemPID/Joint 3/MATLAB Function ==
  data: ddtheta1 input; MTau3 output; theta2 input; ddtheta2 input; theta3 input; theta1 input; ddtheta3 input
function MTau3  = MassMatrix(ddtheta1,theta2,ddtheta2, theta3, theta1,ddtheta3)

MTau3=0.000032669184954733717964837201853562*ddtheta1*cos(theta2 + theta3 + 1.569333479860983395711863672254) - ddtheta2*(0.00035112762269531248284989977115345*cos(2.0*theta2 - 0.069813170079773183076947630739545*theta1 + 2.0*theta3) + 0.00035112762269531248284989977115345*cos(0.069813170079773183076947630739545*theta1 + 2.0*theta2 + 2.0*theta3) - 0.0011037232959375000134610855795358*cos(2.0*theta2 + theta3) + 0.00055186164796875000673054278976792*cos(theta3 - 0.069813170079773183076947630739545*theta1) + 0.00055186164796875000673054278976792*cos(0.069813170079773183076947630739545*theta1 + theta3) + 0.00055186164796875000673054278976792*cos(2.0*theta2 - 0.069813170079773183076947630739545*theta1 + theta3) + 0.00055186164796875000673054278976792*cos(0.069813170079773183076947630739545*theta1 + 2.0*theta2 + theta3) + 0.00070225524539062496569979954230689*cos(0.069813170079773183076947630739545*theta1) - 0.0011037232959375000134610855795358*cos(theta3) - 0.00070225524539062496569979954230689*cos(2.0*theta2 + 2.0*theta3) - 0.0069535131453906254619945492834177) - ddtheta3*(0.00035112762269531248284989977115345*cos(2.0*theta2 - 0.069813170079773183076947630739544*theta1 + 2.0*theta3) + 0.00035112762269531248284989977115345*cos(0.069813170079773183076947630739544*theta1 + 2.0*theta2 + 2.0*theta3) - 0.00070225524539062496569979954230689*cos(2*theta2 + 2*theta3) + 0.00070225524539062496569979954230689*cos(0.069813170079773183076947630739544*theta1) - 0.0069535131453906254619945492834177);
end

== matlab function ControlSystemPID/MATLAB Function ==
  data: th1_0 input; theta1 output; th1_f input; th2_0 input; th2_f input; th3_0 input; th3_f input; t input; dtheta1 output; ddtheta1 output; theta2 output; dtheta2 output; ddtheta2 output; theta3 output; dtheta3 output; ddtheta3 output
function [theta1,dtheta1,ddtheta1,theta2,dtheta2,ddtheta2,theta3,dtheta3,ddtheta3]= trac(th1_0,th1_f,th2_0,th2_f,th3_0,th3_f,t)

tf=3;
a01=th1_0;
a11=0;
a21=(3/tf^2)*(th1_f-th1_0);
a31=-(2/tf^3)*(th1_f-th1_0);
theta1=a01+a11*t+a21*t^2+a31*t^3
dtheta1=a11+2*a21*t+3*a31*t^2;
ddtheta1=2*a21+6*a31*t;

 

a02=th2_0;
a12=0;
a22=(3/tf^2)*(th2_f-th2_0);
a32=-(2/tf^3)*(th2_f-th2_0);
theta2=a02+a12*t+a22*t^2+a32*t^3
dtheta2=a12+2*a22*t+3*a32*t^2;
ddtheta2=2*a22+6*a32*t;

a03=th2_0;
a13=0;
a23=(3/tf^2)*(th3_f-th3_0);
a33=-(2/tf^3)*(th3_f-th3_0);
theta3=a03+a13*t+a23*t^2+a33*t^3
dtheta3=a13+2*a23*t+3*a33*t^2;
ddtheta3=2*a23+6*a33*t;


if tf<t
theta1=a01+a11*tf+a21*tf^2+a31*tf^3
dtheta1=a11+2*a21*tf+3*a31*tf^2;
ddtheta1=0;

theta2=a02+a12*tf+a22*tf^2+a32*tf^3
dtheta2=a12+2*a22*tf+3*a32*tf^2;
ddtheta2=0;

theta3=a03+a13*tf+a23*tf^2+a33*tf^3
dtheta3=a13+2*a23*tf+3*a33*tf^2;
ddtheta3=0;

%theta3=th3_f;
%dtheta3=0;
%ddtheta3=0;
end

== matlab function ControlSystemPID/Joint 2/MATLAB Function ==
  data: ddtheta1 input; MTau2 output; theta2 input; ddtheta2 input; theta3 input; theta1 input; ddtheta3 input
function MTau2  = MassMatrix(ddtheta1,theta2,ddtheta2, theta3, theta1,ddtheta3)

MTau2=ddtheta2*(0.0026084163692907500094186890038372*cos(2.0*theta2) - 0.0033106716146813750835387057946946*cos(0.069813170079773183076947630739545*theta1) + 0.0022074465918750000269221711590717*cos(theta3) + 0.00070225524539062496569979954230689*cos(2.0*theta2)*cos(2.0*theta3) - 0.0026084163692907500094186890038372*cos(2.0*theta2)*cos(0.069813170079773183076947630739545*theta1) - 0.00070225524539062496569979954230689*sin(2.0*theta2)*sin(2.0*theta3) + 0.0022074465918750000269221711590717*cos(2.0*theta2)*cos(theta3) - 0.0022074465918750000269221711590717*cos(0.069813170079773183076947630739545*theta1)*cos(theta3) - 0.0022074465918750000269221711590717*sin(2.0*theta2)*sin(theta3) - 0.0022074465918750000269221711590717*cos(2.0*theta2)*cos(0.069813170079773183076947630739545*theta1)*cos(theta3) + 0.0022074465918750000269221711590717*cos(0.069813170079773183076947630739545*theta1)*sin(2.0*theta2)*sin(theta3) - 0.00070225524539062496569979954230689*cos(2.0*theta2)*cos(2.0*theta3)*cos(0.069813170079773183076947630739545*theta1) + 0.00070225524539062496569979954230689*cos(0.069813170079773183076947630739545*theta1)*sin(2.0*theta2)*sin(2.0*theta3) + 0.017238061144681376957166207830596) + ddtheta3*(0.0011037232959375000134610855795358*cos(theta3) - 0.00070225524539062496569979954230689*cos(0.069813170079773183076947630739545*theta1) + 0.00070225524539062496569979954230689*cos(2.0*theta2)*cos(2.0*theta3) - 0.00070225524539062496569979954230689*sin(2.0*theta2)*sin(2.0*theta3) + 0.0011037232959375000134610855795358*cos(2.0*theta2)*cos(theta3) - 0.0011037232959375000134610855795358*cos(0.069813170079773183076947630739545*theta1)*cos(theta3) - 0.0011037232959375000134610855795358*sin(2.0*theta2)*sin(theta3) - 0.0011037232959375000134610855795358*cos(2.0*theta2)*cos(0.069813170079773183076947630739545*theta1)*cos(theta3) + 0.0011037232959375000134610855795358*cos(0.069813170079773183076947630739545*theta1)*sin(2.0*theta2)*sin(theta3) - 0.00070225524539062496569979954230689*cos(2.0*theta2)*cos(2.0*theta3)*cos(0.069813170079773183076947630739545*theta1) + 0.00070225524539062496569979954230689*cos(0.069813170079773183076947630739545*theta1)*sin(2.0*theta2)*sin(2.0*theta3) + 0.0069535131453906254619945492834177) + ddtheta1*(0.000032669184954733717964837201853562*cos(theta2 + theta3 + 1.569333479860983395711863672254) - 0.000017807919999999997375493554496728*sin(theta2));
end

== matlab function ControlSystemPID/Joint 2/MATLAB Function1 ==
  data: theta1 input; VGTau2 output; dtheta1 input; theta2 input; dtheta2 input; theta3 input; dtheta3 input
function VGTau2 = VelocityGravity(theta1,dtheta1,theta2,dtheta2, theta3,dtheta3)
g =-9.82;
V=0.00028211581843749967577969495202694*dtheta1^2*sin(2.0*theta2 + 2.0*theta3) - 0.000000071470000000000004039742986742395*dtheta1^2*cos(2.0*theta2 + 2.0*theta3) - 0.0011037232959375000134610855795358*dtheta3^2*sin(theta3) - 0.00070225524539062496569979954230689*dtheta2^2*sin(2.0*theta2 + 2.0*theta3) - 0.00070225524539062496569979954230689*dtheta3^2*sin(2.0*theta2 + 2.0*theta3) - 0.0013042081846453750047093445019186*dtheta2^2*sin(0.069813170079773183076947630739544*theta1 - 2.0*theta2) + 0.0013042081846453750047093445019186*dtheta2^2*sin(0.069813170079773183076947630739544*theta1 + 2.0*theta2) + 0.00035112762269531248284989977115345*dtheta2^2*sin(2.0*theta2 - 0.069813170079773183076947630739544*theta1 + 2.0*theta3) + 0.00035112762269531248284989977115345*dtheta2^2*sin(0.069813170079773183076947630739544*theta1 + 2.0*theta2 + 2.0*theta3) + 0.00035112762269531248284989977115345*dtheta3^2*sin(2.0*theta2 - 0.069813170079773183076947630739544*theta1 + 2.0*theta3) + 0.00035112762269531248284989977115345*dtheta3^2*sin(0.069813170079773183076947630739544*theta1 + 2.0*theta2 + 2.0*theta3) - 0.0088297863675000001076886846362868*dtheta1^2*sin(2.0*theta2 + theta3) - 0.0022074465918750000269221711590717*dtheta2^2*sin(2.0*theta2 + theta3) - 0.0011037232959375000134610855795358*dtheta3^2*sin(2.0*theta2 + theta3) + 0.00055186164796875000673054278976792*dtheta3^2*sin(0.069813170079773183076947630739544*theta1 + theta3) + 0.0011037232959375000134610855795358*dtheta2^2*sin(2.0*theta2 - 0.069813170079773183076947630739544*theta1 + theta3) + 0.0011037232959375000134610855795358*dtheta2^2*sin(0.069813170079773183076947630739544*theta1 + 2.0*theta2 + theta3) + 0.00055186164796875000673054278976792*dtheta3^2*sin(2.0*theta2 - 0.069813170079773183076947630739544*theta1 + theta3) + 0.00055186164796875000673054278976792*dtheta3^2*sin(0.069813170079773183076947630739544*theta1 + 2.0*theta2 + theta3) + 0.000011588219999999999987663756861878*dtheta1^2*cos(2.0*theta2) - 0.0066126016171630004614190312395294*dtheta1^2*sin(2.0*theta2) - 0.0026084163692907500094186890038372*dtheta2^2*sin(2.0*theta2) - 0.00055186164796875000673054278976792*dtheta3^2*sin(0.069813170079773183076947630739544*theta1 - theta3) - 0.0022074465918750000269221711590717*dtheta2*dtheta3*sin(theta3) - 0.0014045104907812499313995990846138*dtheta2*dtheta3*sin(2.0*theta2 + 2.0*theta3) + 0.000091050907814079786155997409125007*dtheta1*dtheta2*sin(0.069813170079773183076947630739544*theta1 - 2.0*theta2) + 0.000091050907814079786155997409125007*dtheta1*dtheta2*sin(0.069813170079773183076947630739544*theta1 + 2.0*theta2) - 0.000024513332442934279188639923319215*dtheta1*dtheta2*sin(2.0*theta2 - 0.069813170079773183076947630739544*theta1 + 2.0*theta3) + 0.000024513332442934279188639923319215*dtheta1*dtheta2*sin(0.069813170079773183076947630739544*theta1 + 2.0*theta2 + 2.0*theta3) - 0.000024513332442934279188639923319215*dtheta1*dtheta3*sin(2.0*theta2 - 0.069813170079773183076947630739544*theta1 + 2.0*theta3) + 0.000024513332442934279188639923319215*dtheta1*dtheta3*sin(0.069813170079773183076947630739544*theta1 + 2.0*theta2 + 2.0*theta3) + 0.00070225524539062496569979954230689*dtheta2*dtheta3*sin(2.0*theta2 - 0.069813170079773183076947630739544*theta1 + 2.0*theta3) + 0.00070225524539062496569979954230689*dtheta2*dtheta3*sin(0.069813170079773183076947630739544*theta1 + 2.0*theta2 + 2.0*theta3) - 0.0022074465918750000269221711590717*dtheta2*dtheta3*sin(2.0*theta2 + theta3) + 0.000077054422180292513467995962894719*dtheta1*dtheta2*sin(0.069813170079773183076947630739544*theta1 + theta3) + 0.000038527211090146256733997981447359*dtheta1*dtheta3*sin(0.069813170079773183076947630739544*theta1 + theta3) + 0.0011037232959375000134610855795358*dtheta2*dtheta3*sin(0.069813170079773183076947630739544*theta1 + theta3) - 0.000077054422180292513467995962894719*dtheta1*dtheta2*sin(2.0*theta2 - 0.069813170079773183076947630739544*theta1 + theta3) + 0.000077054422180292513467995962894719*dtheta1*dtheta2*sin(0.069813170079773183076947630739544*theta1 + 2.0*theta2 + theta3) - 0.000038527211090146256733997981447359*dtheta1*dtheta3*sin(2.0*theta2 - 0.069813170079773183076947630739544*theta1 + theta3) + 0.000038527211090146256733997981447359*dtheta1*dtheta3*sin(0.069813170079773183076947630739544*theta1 + 2.0*theta2 + theta3) + 0.0011037232959375000134610855795358*dtheta2*dtheta3*sin(2.0*theta2 - 0.069813170079773183076947630739544*theta1 + theta3) + 0.0011037232959375000134610855795358*dtheta2*dtheta3*sin(0.069813170079773183076947630739544*theta1 + 2.0*theta2 + theta3) + 0.00023112848051402813068927466488844*dtheta1*dtheta2*sin(0.069813170079773183076947630739544*theta1) + 0.00004902666488586855837727984663843*dtheta1*dtheta3*sin(0.069813170079773183076947630739544*theta1) + 0.000077054422180292513467995962894719*dtheta1*dtheta2*sin(0.069813170079773183076947630739544*theta1 - theta3) + 0.000038527211090146256733997981447359*dtheta1*dtheta3*sin(0.069813170079773183076947630739544*theta1 - theta3) - 0.0011037232959375000134610855795358*dtheta2*dtheta3*sin(0.069813170079773183076947630739544*theta1 - theta3);
G=0.040171912499999996859489925782327*g*cos(theta2 + theta3) + 0.10170991059999999472918119636233*g*cos(theta2);
VGTau2=V+G;
end

== matlab function ControlSystemPID/Joint 3/MATLAB Function1 ==
  data: theta1 input; VGTau3 output; dtheta1 input; theta2 input; dtheta2 input; theta3 input; dtheta3 input
function VGTau3 = VelocityGravity(theta1,dtheta1,theta2,dtheta2, theta3,dtheta3)
g =-9.82;
G=0.040171912499999996859489925782327*g*cos(theta2 + theta3);
V=0.00028211581843749967577969495202694*dtheta1^2*sin(2.0*theta2 + 2.0*theta3) - 0.000000071470000000000004039742986742395*dtheta1^2*cos(2.0*theta2 + 2.0*theta3) - 0.0011037232959375000134610855795358*dtheta3^2*sin(theta3) - 0.00070225524539062496569979954230689*dtheta2^2*sin(2.0*theta2 + 2.0*theta3) - 0.00070225524539062496569979954230689*dtheta3^2*sin(2.0*theta2 + 2.0*theta3) - 0.0013042081846453750047093445019186*dtheta2^2*sin(0.069813170079773183076947630739544*theta1 - 2.0*theta2) + 0.0013042081846453750047093445019186*dtheta2^2*sin(0.069813170079773183076947630739544*theta1 + 2.0*theta2) + 0.00035112762269531248284989977115345*dtheta2^2*sin(2.0*theta2 - 0.069813170079773183076947630739544*theta1 + 2.0*theta3) + 0.00035112762269531248284989977115345*dtheta2^2*sin(0.069813170079773183076947630739544*theta1 + 2.0*theta2 + 2.0*theta3) + 0.00035112762269531248284989977115345*dtheta3^2*sin(2.0*theta2 - 0.069813170079773183076947630739544*theta1 + 2.0*theta3) + 0.00035112762269531248284989977115345*dtheta3^2*sin(0.069813170079773183076947630739544*theta1 + 2.0*theta2 + 2.0*theta3) - 0.0088297863675000001076886846362868*dtheta1^2*sin(2.0*theta2 + theta3) - 0.0022074465918750000269221711590717*dtheta2^2*sin(2.0*theta2 + theta3) - 0.0011037232959375000134610855795358*dtheta3^2*sin(2.0*theta2 + theta3) + 0.00055186164796875000673054278976792*dtheta3^2*sin(0.069813170079773183076947630739544*theta1 + theta3) + 0.0011037232959375000134610855795358*dtheta2^2*sin(2.0*theta2 - 0.069813170079773183076947630739544*theta1 + theta3) + 0.0011037232959375000134610855795358*dtheta2^2*sin(0.069813170079773183076947630739544*theta1 + 2.0*theta2 + theta3) + 0.00055186164796875000673054278976792*dtheta3^2*sin(2.0*theta2 - 0.069813170079773183076947630739544*theta1 + theta3) + 0.00055186164796875000673054278976792*dtheta3^2*sin(0.069813170079773183076947630739544*theta1 + 2.0*theta2 + theta3) + 0.000011588219999999999987663756861878*dtheta1^2*cos(2.0*theta2) - 0.0066126016171630004614190312395294*dtheta1^2*sin(2.0*theta2) - 0.0026084163692907500094186890038372*dtheta2^2*sin(2.0*theta2) - 0.00055186164796875000673054278976792*dtheta3^2*sin(0.069813170079773183076947630739544*theta1 - theta3) - 0.0022074465918750000269221711590717*dtheta2*dtheta3*sin(theta3) - 0.0014045104907812499313995990846138*dtheta2*dtheta3*sin(2.0*theta2 + 2.0*theta3) + 0.000091050907814079786155997409125007*dtheta1*dtheta2*sin(0.069813170079773183076947630739544*theta1 - 2.0*theta2) + 0.000091050907814079786155997409125007*dtheta1*dtheta2*sin(0.069813170079773183076947630739544*theta1 + 2.0*theta2) - 0.000024513332442934279188639923319215*dtheta1*dtheta2*sin(2.0*theta2 - 0.069813170079773183076947630739544*theta1 + 2.0*theta3) + 0.000024513332442934279188639923319215*dtheta1*dtheta2*sin(0.069813170079773183076947630739544*theta1 + 2.0*theta2 + 2.0*theta3) - 0.000024513332442934279188639923319215*dtheta1*dtheta3*sin(2.0*theta2 - 0.069813170079773183076947630739544*theta1 + 2.0*theta3) + 0.000024513332442934279188639923319215*dtheta1*dtheta3*sin(0.069813170079773183076947630739544*theta1 + 2.0*theta2 + 2.0*theta3) + 0.00070225524539062496569979954230689*dtheta2*dtheta3*sin(2.0*theta2 - 0.069813170079773183076947630739544*theta1 + 2.0*theta3) + 0.00070225524539062496569979954230689*dtheta2*dtheta3*sin(0.069813170079773183076947630739544*theta1 + 2.0*theta2 + 2.0*theta3) - 0.0022074465918750000269221711590717*dtheta2*dtheta3*sin(2.0*theta2 + theta3) + 0.000077054422180292513467995962894719*dtheta1*dtheta2*sin(0.069813170079773183076947630739544*theta1 + theta3) + 0.000038527211090146256733997981447359*dtheta1*dtheta3*sin(0.069813170079773183076947630739544*theta1 + theta3) + 0.0011037232959375000134610855795358*dtheta2*dtheta3*sin(0.069813170079773183076947630739544*theta1 + theta3) - 0.000077054422180292513467995962894719*dtheta1*dtheta2*sin(2.0*theta2 - 0.069813170079773183076947630739544*theta1 + theta3) + 0.000077054422180292513467995962894719*dtheta1*dtheta2*sin(0.069813170079773183076947630739544*theta1 + 2.0*theta2 + theta3) - 0.000038527211090146256733997981447359*dtheta1*dtheta3*sin(2.0*theta2 - 0.069813170079773183076947630739544*theta1 + theta3) + 0.000038527211090146256733997981447359*dtheta1*dtheta3*sin(0.069813170079773183076947630739544*theta1 + 2.0*theta2 + theta3) + 0.0011037232959375000134610855795358*dtheta2*dtheta3*sin(2.0*theta2 - 0.069813170079773183076947630739544*theta1 + theta3) + 0.0011037232959375000134610855795358*dtheta2*dtheta3*sin(0.069813170079773183076947630739544*theta1 + 2.0*theta2 + theta3) + 0.00023112848051402813068927466488844*dtheta1*dtheta2*sin(0.069813170079773183076947630739544*theta1) + 0.00004902666488586855837727984663843*dtheta1*dtheta3*sin(0.069813170079773183076947630739544*theta1) + 0.000077054422180292513467995962894719*dtheta1*dtheta2*sin(0.069813170079773183076947630739544*theta1 - theta3) + 0.000038527211090146256733997981447359*dtheta1*dtheta3*sin(0.069813170079773183076947630739544*theta1 - theta3) - 0.0011037232959375000134610855795358*dtheta2*dtheta3*sin(0.069813170079773183076947630739544*theta1 - theta3);
VGTau3=V+G;
end

== matlab function ControlSystemPID/Joint 2/MATLAB Function2 ==
  data: ddtheta input; output output; Verror input; Perror input; PiError input; Kp input; Kv input; Ki input
function output = PID(ddtheta, Verror, Perror, PiError,Kp,Kv,Ki)

output = ddtheta+Kv*Verror+Kp*Perror+Ki*PiError;
